simulink model "spaceVector"  (R2018a)
settings: Solver=VariableStepDiscrete  StartTime=0.0  StopTime=0.5  FixedStep=1e-5  RelTol=1e-3
libraries: powerlib x23
settings Model: Creator=enes_  LastModifiedBy=enes_

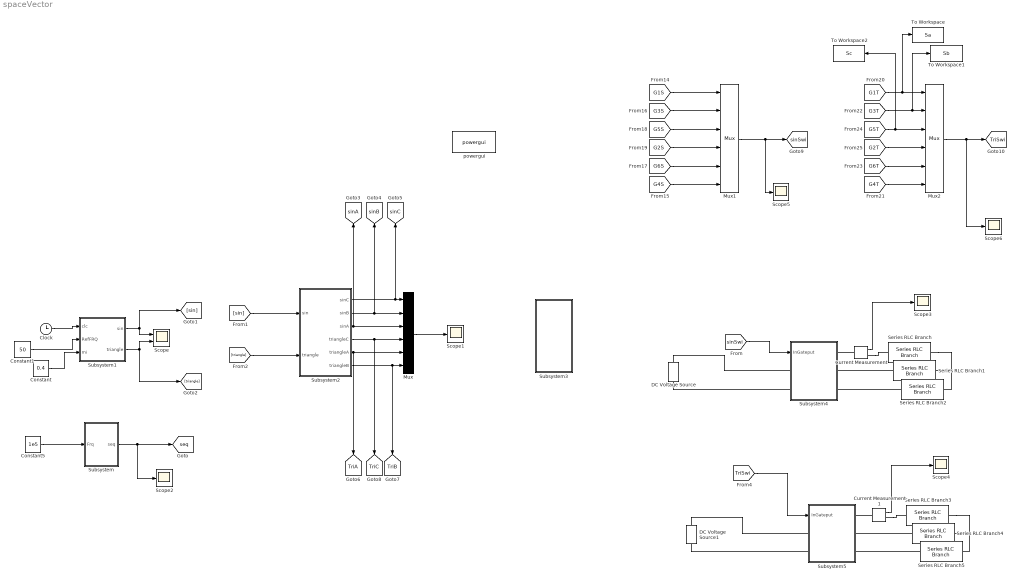
== system spaceVector ==
  Clock : Clock
  Constant : Constant  Value=0.4
  Constant1 : Constant  Value=50
  Constant5 : Constant  Value=1e5
  Current Measurement : powerlib/Measurements/Current Measurement  PhasorSimulation=off  OutputType=Complex  PSBequivalent=0
  Current Measurement1 : powerlib/Measurements/Current Measurement  PhasorSimulation=off  OutputType=Complex  PSBequivalent=0
  DC Voltage Source : powerlib/Electrical Sources/DC Voltage Source  Amplitude=500  Measurements=None
  DC Voltage Source1 : powerlib/Electrical Sources/DC Voltage Source  Amplitude=500  Measurements=None
  Mux : Mux  Inputs=6
  Mux1 : Mux  Inputs=6
  Mux2 : Mux  Inputs=6
  Scope : Scope  NumInputPorts=2
  Scope{1..6} (6 alike) : Scope
  Series RLC Branch{,1..5} (6 alike) : powerlib/Elements/Series RLC Branch  LConnTagsString=__new0  RConnTagsString=__new0  BranchType=RL  Resistance=0.1  Inductance=1  SetiL0=off  InitialCurrent=0  Capacitance=1e-6  Setx0=off  InitialVoltage=0  Measurements=None
  Subsystem : Subsystem
  Subsystem1 : Subsystem
  Subsystem2 : Subsystem
  Subsystem3 : Subsystem
  Subsystem4 : Subsystem
  Subsystem5 : Subsystem
  To Workspace : ToWorkspace  VariableName=Sa  SaveFormat=Timeseries  SampleTime=-1
  To Workspace1 : ToWorkspace  VariableName=Sb  SaveFormat=Timeseries  SampleTime=-1
  To Workspace2 : ToWorkspace  VariableName=Sc  SaveFormat=Timeseries  SampleTime=-1
  powergui : powerlib/powergui  Priority=1  SimulationMode=Discrete  SampleTime=1e-7  frequency=60  Iterations=50  frequencyindice=0  Pbase=100e6  ErrMax=1e-4  UnitsV=kV  UnitsW=MW  buscounter=0  FunctionMessages=off  echomessages=off  EnableUseOfTLC=off  CurrentSourceSwitches=off  DisableSnubberDevices=off  DisableRonSwitches=off  DisableVfSwitches=off  DisplayEquations=off  SolverType=Tustin/Backward Euler (TBE)  Interpol=off  ExternalGateDelay=off  methode=off  Ts=100  x0status=blocks  SPID=on  SwTol=0  HookPort=off  RestoreLinks=warning  ResistiveCurrentMeasurement=off  Frange=[0:2:500]  Ylog=off  Xlog=on  ShowGrid=off  save=off  variable=ZData  structure=0  ZoomFFT=off  StartTime=0.0  cycles=1  DisplayStyle=1  fundamental=60  FreqAxis=off  MaxFrequency=1000  frequencyindicesteady=1  RmsSteady=1  display=off
  tag scope: TriA=global, TriB=global, TriC=global, TriSwi=global, seq=global, sinA=global, sinB=global, sinC=global, sinSwi=global
  wires:
  Constant5/1 -> Subsystem/1(Frq)
  Subsystem/1("seq ") -> Scope2/1, [seq]
  Subsystem1/2(triangle) -> [triangle], Scope/2
  Subsystem1/1(sin) -> [sin], Scope/1
  Clock/1 -> Subsystem1/1(clc)
  Constant1/1 -> Subsystem1/2(RefFRQ)
  [sin] -> Subsystem2/1(sin)
  [triangle] -> Subsystem2/2(triangle)
  Subsystem2/5(triangleA) -> Mux/5, [TriA]
  Subsystem2/4(triangleC) -> [TriC], Mux/4
  Subsystem2/2(sinB) -> Mux/2, [sinB]
  Mux/1 -> Scope1/1
  Subsystem2/3(sinA) -> Mux/3, [sinA]
  Subsystem2/1(sinC) -> [sinC], Mux/1
  Subsystem2/6(triangleB) -> [TriB], Mux/6
  [G3S] -> Mux1/2
  [G1S] -> Mux1/1
  [G5S] -> Mux1/3
  [G2S] -> Mux1/4
  [G6S] -> Mux1/5
  [G4S] -> Mux1/6
  Mux1/1 -> Scope5/1, [sinSwi]
  [sinSwi] -> Subsystem4/1(InGateput)
  Current Measurement/1 -> Scope3/1
  [TriSwi] -> Subsystem5/1(InGateput)
  Current Measurement1/1 -> Scope4/1
  [G3T] -> To Workspace1/1, Mux2/2
  [G5T] -> To Workspace2/1, Mux2/3
  [G2T] -> Mux2/4
  [G6T] -> Mux2/5
  [G4T] -> Mux2/6
  Mux2/1 -> Scope6/1, [TriSwi]
  Constant/1 -> Subsystem1/3(mi)
  [G1T] -> To Workspace/1, Mux2/1
  connections:
  DC Voltage Source/RConn1 -- Subsystem4/LConn1
  DC Voltage Source/LConn1 -- Subsystem4/LConn2
  Series RLC Branch1/LConn1 -- Subsystem4/RConn2
  Series RLC Branch2/LConn1 -- Subsystem4/RConn3
  Series RLC Branch/RConn1 -- Series RLC Branch2/RConn1 -- Series RLC Branch1/RConn1
  Current Measurement/LConn1 -- Subsystem4/RConn1
  Current Measurement/RConn1 -- Series RLC Branch/LConn1
  Series RLC Branch4/RConn1 -- Series RLC Branch3/RConn1 -- Series RLC Branch5/RConn1
  Series RLC Branch5/LConn1 -- Subsystem5/RConn3
  Series RLC Branch4/LConn1 -- Subsystem5/RConn2
  Current Measurement1/RConn1 -- Series RLC Branch3/LConn1
  Current Measurement1/LConn1 -- Subsystem5/RConn1
  DC Voltage Source1/RConn1 -- Subsystem5/LConn1
  DC Voltage Source1/LConn1 -- Subsystem5/LConn2

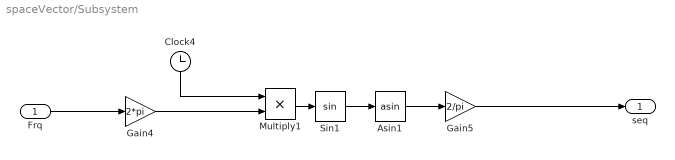
== system spaceVector/Subsystem ==
  Frq : Inport
  Asin1 : Trigonometry  Operator=asin
  Clock4 : Clock
  Gain4 : Gain  Gain=2*pi
  Gain5 : Gain  Gain=2/pi
  Multiply1 : Product
  Sin1 : Trigonometry
  "seq " : Outport
  wires:
  Frq/1 -> Gain4/1
  Asin1/1 -> Gain5/1
  Gain5/1 -> "seq "/1
  Multiply1/1 -> Sin1/1
  Sin1/1 -> Asin1/1
  Gain4/1 -> Multiply1/2
  Clock4/1 -> Multiply1/1

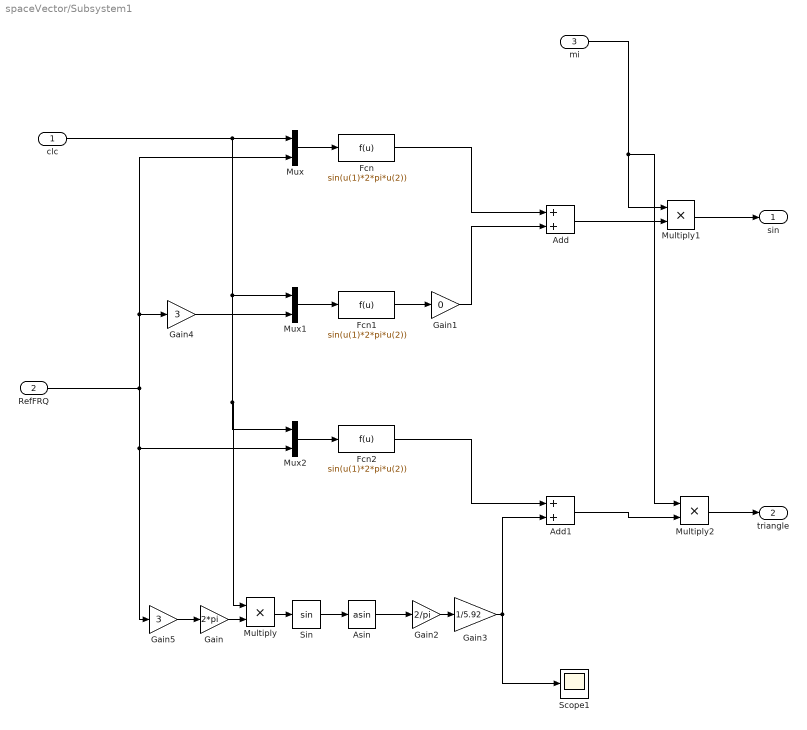
== system spaceVector/Subsystem1 ==
  clc : Inport
  RefFRQ : Inport  Port=2
  mi : Inport  Port=3
  Add : Sum
  Add1 : Sum
  Asin : Trigonometry  Operator=asin
  Fcn : Fcn  Expr=sin(u(1)*2*pi*u(2))
  Fcn1 : Fcn  Expr=sin(u(1)*2*pi*u(2))
  Fcn2 : Fcn  Expr=sin(u(1)*2*pi*u(2))
  Gain : Gain  Gain=2*pi
  Gain1 : Gain  Gain=0
  Gain2 : Gain  Gain=2/pi
  Gain3 : Gain  Gain=1/5.92
  Gain4 : Gain  Gain=3
  Gain5 : Gain  Gain=3
  Multiply : Product
  Multiply1 : Product
  Multiply2 : Product
  Mux : Mux  Inputs=2
  Mux1 : Mux  Inputs=2
  Mux2 : Mux  Inputs=2
  Scope1 : Scope
  Sin : Trigonometry
  sin : Outport
  triangle : Outport  Port=2
  wires:
  Fcn1/1 -> Gain1/1
  Mux2/1 -> Fcn2/1
  Mux1/1 -> Fcn1/1
  Mux/1 -> Fcn/1
  Asin/1 -> Gain2/1
  clc/1 -> Multiply/1, Mux2/1, Mux1/1, Mux/1
  Fcn/1 -> Add/1
  Sin/1 -> Asin/1
  Gain/1 -> Multiply/2
  Gain2/1 -> Gain3/1
  Gain1/1 -> Add/2
  Multiply/1 -> Sin/1
  Gain4/1 -> Mux1/2
  Fcn2/1 -> Add1/1
  Gain3/1 -> Scope1/1, Add1/2
  RefFRQ/1 -> Mux/2, Gain4/1, Gain5/1, Mux2/2
  Gain5/1 -> Gain/1
  Add/1 -> Multiply1/2
  Multiply1/1 -> sin/1
  Add1/1 -> Multiply2/2
  Multiply2/1 -> triangle/1
  mi/1 -> Multiply2/1, Multiply1/1

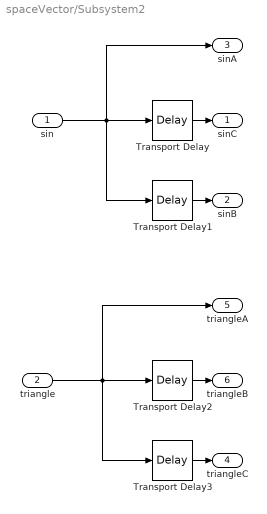
== system spaceVector/Subsystem2 ==
  sin : Inport
  triangle : Inport  Port=2
  Transport Delay : TransportDelay  DelayTime=(1/150)
  Transport Delay1 : TransportDelay  DelayTime=2/150
  Transport Delay2 : TransportDelay  DelayTime=(1/150)
  Transport Delay3 : TransportDelay  DelayTime=2/150
  sinC : Outport
  sinB : Outport  Port=2
  sinA : Outport  Port=3
  triangleC : Outport  Port=4
  triangleA : Outport  Port=5
  triangleB : Outport  Port=6
  wires:
  Transport Delay1/1 -> sinB/1
  sin/1 -> sinA/1, Transport Delay1/1, Transport Delay/1
  Transport Delay2/1 -> triangleB/1
  triangle/1 -> triangleA/1, Transport Delay3/1, Transport Delay2/1
  Transport Delay3/1 -> triangleC/1
  Transport Delay/1 -> sinC/1

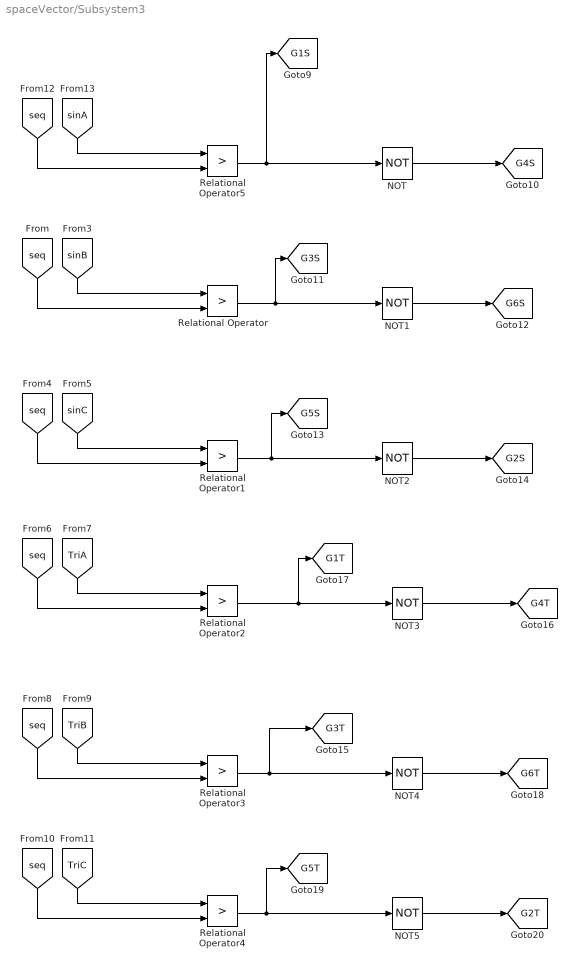
== system spaceVector/Subsystem3 ==
  NOT{,1..5} (6 alike) : Logic  Operator=NOT  AllPortsSameDT=off  OutDataTypeStr=boolean
  Relational Operator{,1..5} (6 alike) : RelationalOperator  Operator=>  OutDataTypeStr=boolean  RndMeth=Simplest
  tag scope: G1S=global, G1T=global, G2S=global, G2T=global, G3S=global, G3T=global, G4S=global, G4T=global, G5S=global, G5T=global, G6S=global, G6T=global
  wires:
  [sinC] -> Relational Operator1/1
  [TriB] -> Relational Operator3/1
  NOT3/1 -> [G4T]
  Relational Operator/1 -> [G3S], NOT1/1
  [seq] -> Relational Operator4/2
  [sinB] -> Relational Operator/1
  [TriC] -> Relational Operator4/1
  Relational Operator5/1 -> [G1S], NOT/1
  [seq] -> Relational Operator3/2
  NOT4/1 -> [G6T]
  Relational Operator3/1 -> NOT4/1, [G3T]
  [sinA] -> Relational Operator5/1
  Relational Operator1/1 -> [G5S], NOT2/1
  Relational Operator2/1 -> [G1T], NOT3/1
  [seq] -> Relational Operator5/2
  [seq] -> Relational Operator/2
  Relational Operator4/1 -> [G5T], NOT5/1
  NOT5/1 -> [G2T]
  NOT/1 -> [G4S]
  [seq] -> Relational Operator2/2
  [TriA] -> Relational Operator2/1
  [seq] -> Relational Operator1/2
  NOT1/1 -> [G6S]
  NOT2/1 -> [G2S]

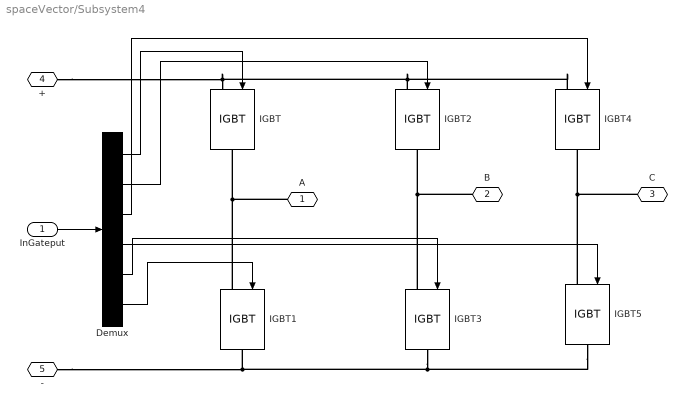
== system spaceVector/Subsystem4 ==
  InGateput : Inport
  Demux : Demux  Outputs=6
  IGBT{,1..5} (6 alike) : powerlib/Power Electronics/IGBT  Ron=0.001  Lon=0  Vf=1  Tf=1e-6  Tt=2e-6  IC=0  Rs=1e5  Cs=inf  Measurements=off
  "A " : PMIOPort  Side=Right
  B : PMIOPort  Port=2  Side=Right
  C : PMIOPort  Port=3  Side=Right
  + : PMIOPort  Port=4  Side=Left
  - : PMIOPort  Port=5  Side=Left
  wires:
  Demux/2 -> IGBT2/1
  InGateput/1 -> Demux/1
  Demux/1 -> IGBT/1
  Demux/5 -> IGBT3/1
  Demux/4 -> IGBT5/1
  Demux/6 -> IGBT1/1
  Demux/3 -> IGBT4/1
  connections:
  IGBT1/RConn1 -- -/RConn1 -- IGBT5/RConn1 -- IGBT3/RConn1
  IGBT/LConn1 -- +/RConn1 -- IGBT4/LConn1 -- IGBT2/LConn1
  IGBT5/LConn1 -- C/RConn1 -- IGBT4/RConn1
  IGBT1/LConn1 -- "A "/RConn1 -- IGBT/RConn1
  IGBT3/LConn1 -- B/RConn1 -- IGBT2/RConn1

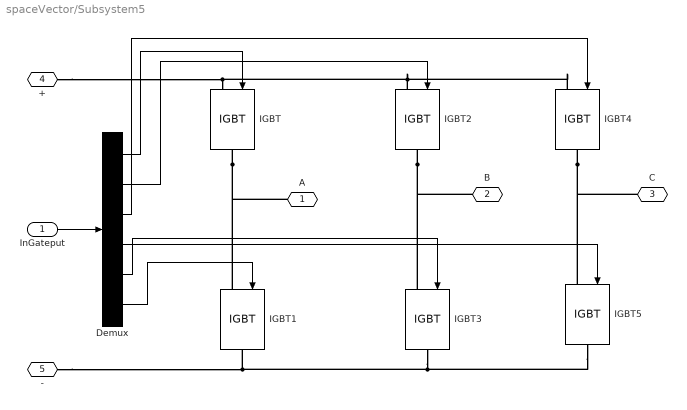
== system spaceVector/Subsystem5 ==
  InGateput : Inport
  Demux : Demux  Outputs=6
  IGBT{,1..5} (6 alike) : powerlib/Power Electronics/IGBT  Ron=0.001  Lon=0  Vf=1  Tf=1e-6  Tt=2e-6  IC=0  Rs=1e5  Cs=inf  Measurements=off
  "A " : PMIOPort  Side=Right
  B : PMIOPort  Port=2  Side=Right
  C : PMIOPort  Port=3  Side=Right
  + : PMIOPort  Port=4  Side=Left
  - : PMIOPort  Port=5  Side=Left
  wires:
  Demux/2 -> IGBT2/1
  InGateput/1 -> Demux/1
  Demux/1 -> IGBT/1
  Demux/5 -> IGBT3/1
  Demux/4 -> IGBT5/1
  Demux/6 -> IGBT1/1
  Demux/3 -> IGBT4/1
  connections:
  IGBT5/RConn1 -- IGBT3/RConn1 -- IGBT1/RConn1 -- -/RConn1
  IGBT4/LConn1 -- IGBT2/LConn1 -- IGBT/LConn1 -- +/RConn1
  IGBT4/RConn1 -- IGBT5/LConn1 -- C/RConn1
  IGBT/RConn1 -- IGBT1/LConn1 -- "A "/RConn1
  IGBT2/RConn1 -- IGBT3/LConn1 -- B/RConn1
